simulink model "superProgramParameterObserving"  (R2014b)
settings: Solver=FixedStepDiscrete  StartTime=0.0  StopTime=10.0  RelTol=1e-3
libraries: c2833xlib x19, c280xlib x7, simulink x1
(part 2 of 2)

== stateflow chart superProgramParameterObserving/stackerController ==
  state stateOne [parallel]
    settings: executionOrder=10
    state storeValue
      entry: lightBarrierTriggeredValue = lightBarrierCrossed;
      colorSensorTriggeredValue = colorSensor;
    state idle
    state start
      entry: lightBarrierTriggeredValue = false;
      colorSensorTriggeredValue = uint16(9999);
    state wait
    stateOne.idle -> storeValue : after(0.01,msec)
    (default) -> stateOne.start
    stateOne.start -> stateOne.idle
    wait -> stateOne.idle
    storeValue -> wait : after(0.01,msec)
  state startingSequence [parallel]
    settings: executionOrder=1
    state prepareStacker
      entry:
      stackerMode = int16(0);
      speedCenterPivotTable = uint16(0);
      directionCenterPivotTable = true;
      speedTowerShifter = uint16(0);
      directionTowerShifter = true;
      speedDoorOpener = uint16(75);
      directionDoorOpener = false;
      paternosterSpeed_controller.setPaternosterSpeed(uint16(0));
      directionPaternoster = true;
      speedKicker = uint16(0);
      directionKicker = true;
      speedTipper = uint16(0);
      directionTipper = true;
      enableCounter;
      state prepareTipper [parallel]
        settings: executionOrder=1
        state tipperPreparation
          entry: directionTipper = true;
          speedTipper = tipperSpeed;
        state stopKickerInStartingPosition
          entry: speedTipper = uint16(0);
        (default) -> startingSequence.prepareStacker.prepareTipper.tipperPreparation
        startingSequence.prepareStacker.prepareTipper.tipperPreparation -> stopKickerInStartingPosition : [innerTipperButton == true]
      state prepareKicker [parallel]
        settings: executionOrder=2
        state startKickerMovement
          entry: speedKicker = uint16(100);
          directionKicker = true;
        state stopKickerMovement
          entry: speedKicker = uint16(0);
        startingSequence.prepareStacker.prepareKicker.startKickerMovement -> startingSequence.prepareStacker.prepareKicker.stopKickerMovement : [innerKickerButton == true]
        (default) -> startingSequence.prepareStacker.prepareKicker.startKickerMovement
      state shiftStackerAndOpenDoor [parallel]
        settings: executionOrder=3
        state blockTowerIdle
        state shiftTowerForwards
          entry: speedDoorOpener = uint16(0);
          directionTowerShifter = false;
          speedTowerShifter = towerShifterSpeed;
        state stopOpeningDoor
          entry: speedDoorOpener = uint16(0);
        state stopTowerShifting
          entry: speedTowerShifter = uint16(0);
          directionTowerShifter = true;
        state openDoor
          entry: directionDoorOpener = true;
          speedDoorOpener = uint16(70);
        blockTowerIdle -> shiftTowerForwards : [towerShifterButton == true]
        (default) -> blockTowerIdle
        shiftTowerForwards -> startingSequence.prepareStacker.shiftStackerAndOpenDoor.stopTowerShifting : [towerShifterButton == false]
        openDoor -> startingSequence.prepareStacker.shiftStackerAndOpenDoor.stopOpeningDoor : [towerShifterButton == false]
        startingSequence.prepareStacker.shiftStackerAndOpenDoor.stopTowerShifting -> openDoor : [towerShifterButton == true]
        startingSequence.prepareStacker.shiftStackerAndOpenDoor.stopOpeningDoor -> openDoor : [towerShifterButton == true]
      state emptyTipper [parallel]
        settings: executionOrder=4
        state wait_1
        state moveTipperIn
          entry: directionTipper = true;
        state tipperIdle
        state moveTipperOut
          entry: directionTipper = false;
          speedTipper = tipperSpeed;
        state wait_2
        (default) -> startingSequence.prepareStacker.emptyTipper.tipperIdle
        startingSequence.prepareStacker.emptyTipper.tipperIdle -> wait_1 : [[outerTipperButton == true] && [innerTipperButton == true]]
        wait_1 -> moveTipperOut : after(1300,msec)
        moveTipperOut -> moveTipperIn : [outerTipperButton == true]
        wait_2 -> startingSequence.prepareStacker.emptyTipper.tipperIdle : after(1300,msec)
        moveTipperIn -> moveTipperOut [order 2] : [innerTipperButton == true]
        moveTipperIn -> wait_2 [order 1] : [[outerTipperButton == true] && [innerTipperButton == true]]
    state operationMode
    state waitingForButtonRelaseToStartSuperProgram
    (default) -> prepareStacker
    prepareStacker -> waitingForButtonRelaseToStartSuperProgram : [powerButton == true]
    waitingForButtonRelaseToStartSuperProgram -> operationMode : [powerButton == false] {send(sorting.START); send(timer.START);}
  state timer [parallel]
    settings: executionOrder=2
    state startReturningBlocksFromRecervoir
      entry: send(sorting.STARTRESORTING);
    state start
    state inactive
    inactive -> startReturningBlocksFromRecervoir : after(latestPointInTimeToAcceptBlockDelivery,sec)
    (default) -> timer.start
    timer.start -> inactive : START
  state statusLED [parallel]
    settings: executionOrder=7
    state LED_1 [parallel]
      settings: executionOrder=1
      state off
        entry: statusLED_1 = false;
      state flash
        entry: statusLED_1 = true;
      state on
        entry: statusLED_1 = true;
      (default) -> statusLED.LED_1.off
      statusLED.LED_1.off -> statusLED.LED_1.on [order 1] : ON
      statusLED.LED_1.on -> statusLED.LED_1.off : OFF
      statusLED.LED_1.flash -> statusLED.LED_1.off : after(300,msec)
      statusLED.LED_1.off -> statusLED.LED_1.flash [order 2] : FLASH
    state LED_2 [parallel]
      settings: executionOrder=2
      state off
        entry: statusLED_2 = false;
      state flash
        entry: statusLED_2 = true;
      state on
        entry: statusLED_2 = true;
      (default) -> statusLED.LED_2.off
      statusLED.LED_2.off -> statusLED.LED_2.on [order 1] : ON
      statusLED.LED_2.on -> statusLED.LED_2.off : OFF
      statusLED.LED_2.flash -> statusLED.LED_2.off : after(300,msec)
      statusLED.LED_2.off -> statusLED.LED_2.flash [order 2] : FLASH
    state LED_3 [parallel]
      settings: executionOrder=3
      state off
        entry: statusLED_3 = false;
      state flash
        entry: statusLED_3 = true;
      state on
        entry: statusLED_3 = true;
      (default) -> statusLED.LED_3.off
      statusLED.LED_3.off -> statusLED.LED_3.on [order 1] : ON
      statusLED.LED_3.on -> statusLED.LED_3.off : OFF
      statusLED.LED_3.flash -> statusLED.LED_3.off : after(300,msec)
      statusLED.LED_3.off -> statusLED.LED_3.flash [order 2] : FLASH
    state LED_4 [parallel]
      settings: executionOrder=4
      state off
        entry: statusLED_4 = false;
      state flash
        entry: statusLED_4 = true;
      state on
        entry: statusLED_4 = true;
      (default) -> statusLED.LED_4.off
      statusLED.LED_4.off -> statusLED.LED_4.on [order 1] : ON
      statusLED.LED_4.on -> statusLED.LED_4.off : OFF
      statusLED.LED_4.flash -> statusLED.LED_4.off : after(300,msec)
      statusLED.LED_4.off -> statusLED.LED_4.flash [order 2] : FLASH
    state LED_finish [parallel]
      settings: executionOrder=5
      state off
        entry: LED_finish = false;
      state flash
        entry: LED_finish = true;
      state on
        entry: LED_finish = true;
      (default) -> statusLED.LED_finish.off
      statusLED.LED_finish.off -> statusLED.LED_finish.on [order 1] : ON
      statusLED.LED_finish.on -> statusLED.LED_finish.off : OFF
      statusLED.LED_finish.flash -> statusLED.LED_finish.off : after(300,msec)
      statusLED.LED_finish.off -> statusLED.LED_finish.flash [order 2] : FLASH
  state counterFromLightBarrierCrossed [parallel]
    settings: executionOrder=3
    state counter
      (history)
      state start
        entry: count = uint32(0);
      state highLevel
      state lowLevel
        entry: count = count + 1;
      counterFromLightBarrierCrossed.counter.lowLevel -> counterFromLightBarrierCrossed.counter.highLevel : [encoderPaternoster == true]
      (default) -> counterFromLightBarrierCrossed.counter.start
      counterFromLightBarrierCrossed.counter.start -> counterFromLightBarrierCrossed.counter.lowLevel : [encoderPaternoster == true]
      counterFromLightBarrierCrossed.counter.highLevel -> counterFromLightBarrierCrossed.counter.lowLevel : [encoderPaternoster == false]
      counterFromLightBarrierCrossed.counter -> counterFromLightBarrierCrossed.counter.start [order 1] : RESET
    state counting_off
    (default) -> counterFromLightBarrierCrossed.counter
    counterFromLightBarrierCrossed.counting_off -> counterFromLightBarrierCrossed.counter : [counterIsEnabled]
    counterFromLightBarrierCrossed.counter -> counterFromLightBarrierCrossed.counting_off [order 1] : [counterIsDisabled]
  state paternosterSpeed_controller [parallel]
    settings: executionOrder=4
    state moveToLastUnblockedPosition
      entry: directionPaternoster = true;
    state paternosterBlocked_errorRoutine
      entry: disableCounter;
      directionPaternoster = false;
      speedPaternoster = uint16(75);
    state restoreNormalPaternosterMode
    state counter
      entry: speedPaternoster = paternosterSpeed_controller.internalPaternosterSpeed;
      (history)
      state highLevel
      state lowLevel
      paternosterSpeed_controller.counter.lowLevel -> paternosterSpeed_controller.counter.highLevel [order 1] : [encoderPaternoster == true]
      (default) -> paternosterSpeed_controller.counter.lowLevel
      paternosterSpeed_controller.counter.highLevel -> paternosterSpeed_controller.counter.lowLevel [order 1] : [encoderPaternoster == false]
    paternosterSpeed_controller.counter.highLevel -> paternosterBlocked_errorRoutine [order 2] : [after(900,msec) && [paternosterSpeed_controller.internalPaternosterSpeed ~= 0]]
    paternosterBlocked_errorRoutine -> moveToLastUnblockedPosition : after(400,msec)
    moveToLastUnblockedPosition -> restoreNormalPaternosterMode : after(400,msec)
    paternosterSpeed_controller.counter.lowLevel -> paternosterBlocked_errorRoutine [order 2] : [after(900,msec) && [paternosterSpeed_controller.internalPaternosterSpeed ~= 0]]
    restoreNormalPaternosterMode -> paternosterSpeed_controller.counter : /{enableCounter;}
    (default) -> paternosterSpeed_controller.counter
    paternosterSpeed_controller.counter -> paternosterSpeed_controller.counter : UPDATEPATERNOSTERSPEED
  state stackerModeStatusLED_controller [parallel]
    settings: executionOrder=8
    state stackerPreparation
      entry: statusLED.LED_1.FLASH;
      statusLED.LED_2.FLASH;
      statusLED.LED_3.FLASH;
      statusLED.LED_4.FLASH;
    state waitingForFirstDelivery
      entry: statusLED.LED_1.ON;
      statusLED.LED_2.ON;
      statusLED.LED_3.ON;
      statusLED.LED_4.ON;
    state colorSortingFirstDelivery
      entry: statusLED.LED_1.ON;
    state waitingForSecondDelivery
      entry: statusLED.LED_2.ON;
    state changeMode
      entry: statusLED.LED_1.OFF;
      statusLED.LED_2.OFF;
      statusLED.LED_3.OFF;
      statusLED.LED_4.OFF;
    state colorSortingSecondDelivery
      entry: statusLED.LED_3.ON;
    state resorting
      entry: statusLED.LED_4.ON;
    state demolding
      entry: statusLED.LED_1.ON;
      statusLED.LED_2.ON;
      statusLED.LED_3.ON;
      statusLED.LED_4.ON;
    state finish
      entry: statusLED.LED_1.FLASH;
      statusLED.LED_2.FLASH;
      statusLED.LED_3.FLASH;
      statusLED.LED_4.FLASH;
    changeMode -> stackerPreparation [order 1] : [stackerMode == 0]
    stackerPreparation -> changeMode : after(1200,msec)
    changeMode -> stackerModeStatusLED_controller.waitingForFirstDelivery [order 2] : [stackerMode == 1]
    stackerModeStatusLED_controller.waitingForFirstDelivery -> changeMode : [stackerMode ~= 1]
    changeMode -> colorSortingFirstDelivery [order 3] : [stackerMode == 2]
    colorSortingFirstDelivery -> changeMode : [stackerMode ~= 2]
    changeMode -> stackerModeStatusLED_controller.waitingForSecondDelivery [order 6] : [stackerMode ==3]
    stackerModeStatusLED_controller.waitingForSecondDelivery -> changeMode : [stackerMode ~= 3]
    changeMode -> colorSortingSecondDelivery [order 4] : [stackerMode == 4]
    colorSortingSecondDelivery -> changeMode : [stackerMode ~= 4]
    (default) -> changeMode
    stackerModeStatusLED_controller.finish -> changeMode : after(600,msec)
    changeMode -> stackerModeStatusLED_controller.finish [order 8] : [stackerMode == 7]
    stackerModeStatusLED_controller.demolding -> changeMode : [stackerMode ~= 6]
    changeMode -> stackerModeStatusLED_controller.demolding [order 7] : [stackerMode == 6]
    resorting -> changeMode : [stackerMode ~= 5]
    changeMode -> resorting [order 5] : [stackerMode == 5]
  note: stackerModes:
      | 0: stackerPreparation
      | 1: waitingForFirstDelivery
      | 2: colorSortingFirstDelivery
      | 3: waitingForSecondDelivery
      | 4: colorSortingSecondDelivery
      | 5: resorting
      | 6: demolding
      | 7: finish
  state blockCounter [parallel]
    settings: executionOrder=9
    state start
      entry: blueBlocksPassed = uint16(0);
      redBlocksPassed = uint16(0);
    state idle
      entry: totalBlocksPassed = blueBlocksPassed + redBlocksPassed;
    blockCounter.idle -> blockCounter.idle [order 2] : ADDBLUEBLOCK
        | /{blueBlocksPassed = blueBlocksPassed + 1;
        | blueBlocksInRecervoir = blueBlocksInRecervoir + 1;}
    blockCounter.start -> blockCounter.idle
    (default) -> blockCounter.start : {blueBlocksInRecervoir = uint16(0);}
    blockCounter.idle -> blockCounter.idle [order 1] : ADDREDBLOCK
        | /{redBlocksPassed = redBlocksPassed + 1;}
    blockCounter -> blockCounter.start : RESET
  state stateTwo [parallel]
    settings: executionOrder=11
    state start
      entry: stateOne.lightBarrierTriggeredValue = stateOne.lightBarrierTriggeredValue;
      stateOne.colorSensorTriggeredValue = stateOne.colorSensorTriggeredValue;
    state end
      entry: stateOne.lightBarrierTriggeredValue = stateOne.lightBarrierTriggeredValue;
      stateOne.colorSensorTriggeredValue = stateOne.colorSensorTriggeredValue;
    (default) -> stateTwo.start
    stateTwo.start -> end
    end -> stateTwo.start : after(0.01,msec)
  state sorting [parallel]
    settings: executionOrder=6
    state resorting_controller
      entry: counterFromLightBarrierCrossed.counter.RESET;
      stackerMode = int16(5);
      blocksInChute = blocksInChute + abs(blocksInChute) * int16([blocksInChute < 0]);
      blocksToTip = int16(blockCapacityFromTipperToPaternosterIntake) - blocksInChute;
      paternosterSpeed_controller.setPaternosterSpeed(paternosterMaximumSpeed);
      state chuteEnquing_controller [parallel]
        settings: executionOrder=1
        state counterDisabled
        state chuteEnqueuing_controller
          (history)
          state idle
          state signalizeFreeSlotInChute
            exit: resorting_controller.blocksToTip = resorting_controller.blocksToTip + 1;
          sorting.resorting_controller.chuteEnquing_controller.chuteEnqueuing_controller.idle -> signalizeFreeSlotInChute : [lightBarrierCrossed == true]
              | {counterFromLightBarrierCrossed.counter.RESET;
              | send(blockCounter.ADDREDBLOCK);}
          (default) -> sorting.resorting_controller.chuteEnquing_controller.chuteEnqueuing_controller.idle
          signalizeFreeSlotInChute -> sorting.resorting_controller.chuteEnquing_controller.chuteEnqueuing_controller.idle : [lightBarrierCrossed == false]
        (default) -> counterDisabled
        chuteEnqueuing_controller -> counterDisabled : [counterIsDisabled]
        counterDisabled -> chuteEnqueuing_controller : [counterIsEnabled]
      state tipper_controller [parallel]
        settings: executionOrder=2
        state tip
          exit: resorting_controller.blocksToTip = resorting_controller. blocksToTip - 1;
          blockCounter.blueBlocksInRecervoir = blockCounter.blueBlocksInRecervoir - 1;
          state tipperMovement
            state tipperPreparation
              entry: directionTipper = false;
              speedTipper = tipperSpeed;
            state tipperBlocked_errorRoutine
              state waitForResolvingOfBlockage
                entry: speedTipper = uint16(0);
              state removeTipperFromBlockage
                entry: directionTipper = false;
                speedTipper = tipperSpeed;
              removeTipperFromBlockage -> waitForResolvingOfBlockage : [outerTipperButton == true]
              (default) -> removeTipperFromBlockage
            state tipperPush
              entry: directionTipper = true;
            state tipperRemove
              entry: directionTipper = false;
            state tipperIdle
              entry: speedTipper = uint16(0);
            (default) -> sorting.resorting_controller.tipper_controller.tip.tipperMovement.tipperPreparation
            waitForResolvingOfBlockage -> sorting.resorting_controller.tipper_controller.tip.tipperMovement.tipperPreparation : after(300,msec)
            sorting.resorting_controller.tipper_controller.tip.tipperMovement.tipperPreparation -> tipperPush : [outerTipperButton == true]
            tipperPush -> tipperBlocked_errorRoutine [order 2] : after(500,msec)
            tipperPush -> tipperRemove [order 1] : [innerTipperButton == true]
            tipperRemove -> sorting.resorting_controller.tipper_controller.tip.tipperMovement.tipperIdle : [outerTipperButton == true]
          (default) -> tipperMovement
        state tipperIdle
        sorting.resorting_controller.tipper_controller.tipperIdle -> tip : [resorting_controller.blocksToTip > 0]
        (default) -> sorting.resorting_controller.tipper_controller.tipperIdle
        sorting.resorting_controller.tipper_controller.tip.tipperMovement.tipperIdle -> sorting.resorting_controller.tipper_controller.tipperIdle : after(250,msec)
    state colorSorter
      entry: paternosterSpeed_controller.setPaternosterSpeed(paternosterSpeed);
      state counterFromKick [parallel]
        settings: executionOrder=2
        state counter
          (history)
          state start
            entry: count = uint32(0);
          state highLevel
          state lowLevel
            entry: count = count + 1;
          sorting.colorSorter.counterFromKick.counter.lowLevel -> sorting.colorSorter.counterFromKick.counter.highLevel : [encoderPaternoster == true]
          (default) -> sorting.colorSorter.counterFromKick.counter.start
          sorting.colorSorter.counterFromKick.counter.start -> sorting.colorSorter.counterFromKick.counter.lowLevel : [encoderPaternoster == true]
          sorting.colorSorter.counterFromKick.counter.highLevel -> sorting.colorSorter.counterFromKick.counter.lowLevel : [encoderPaternoster == false]
          sorting.colorSorter.counterFromKick.counter -> sorting.colorSorter.counterFromKick.counter.start [order 1] : RESET
        state counting_off
        sorting.colorSorter.counterFromKick.counting_off -> sorting.colorSorter.counterFromKick.counter : [counterIsEnabled]
        (default) -> sorting.colorSorter.counterFromKick.counting_off
        sorting.colorSorter.counterFromKick.counter -> sorting.colorSorter.counterFromKick.counting_off [order 1] : [counterIsDisabled]
      state kicker [parallel]
        settings: executionOrder=1
        state kicker_controller [parallel]
          settings: executionOrder=1
          state kick
            entry: send(colorSorter.counterFromKick.counter.RESET);
            enqueuedBlocksToKick = enqueuedBlocksToKick -1;
            state startKickerMovement
              entry: directionKicker = false;
              speedKicker = uint16(100);
            state stopKickerMovement
              entry: speedKicker = uint16(0);
            state kickerBlocked_errorRoutine
              state dissolveBlockage
                entry: disableCounter;
                paternosterSpeed_controller.setPaternosterSpeed(uint16(70));
                directionPaternoster = false;
              state resumeNormalPaternosterOperatingMode
                exit: enableCounter;
                directionPaternoster = true;
                speedPaternoster = uint16(paternosterSpeed);
              (default) -> sorting.colorSorter.kicker.kicker_controller.kick.kickerBlocked_errorRoutine.dissolveBlockage
              sorting.colorSorter.kicker.kicker_controller.kick.kickerBlocked_errorRoutine.dissolveBlockage -> sorting.colorSorter.kicker.kicker_controller.kick.kickerBlocked_errorRoutine.resumeNormalPaternosterOperatingMode : [outerKickerButton == true]
            sorting.colorSorter.kicker.kicker_controller.kick.startKickerMovement -> sorting.colorSorter.kicker.kicker_controller.kick.stopKickerMovement [order 1] : [outerKickerButton == true]
            (default) -> sorting.colorSorter.kicker.kicker_controller.kick.startKickerMovement
            sorting.colorSorter.kicker.kicker_controller.kick.kickerBlocked_errorRoutine.resumeNormalPaternosterOperatingMode -> sorting.colorSorter.kicker.kicker_controller.kick.stopKickerMovement
            sorting.colorSorter.kicker.kicker_controller.kick.startKickerMovement -> sorting.colorSorter.kicker.kicker_controller.kick.kickerBlocked_errorRoutine [order 2] : after(kickerBlockedTimeout,msec)
          state idle
            entry: speedKicker = uint16(0);
          state reprepareKicker
            state kickerBlocked_errorRoutine
              state dissolveBlockage
                entry: speedKicker = uint16(100);
                directionKicker = false;
              (default) -> sorting.colorSorter.kicker.kicker_controller.reprepareKicker.kickerBlocked_errorRoutine.dissolveBlockage
            state startKickerMovement
              entry: speedKicker = uint16(100);
              directionKicker = true;
            state stopKickerMovement
              entry: speedKicker = uint16(0);
            sorting.colorSorter.kicker.kicker_controller.reprepareKicker.startKickerMovement -> sorting.colorSorter.kicker.kicker_controller.reprepareKicker.kickerBlocked_errorRoutine [order 2] : after(kickerBlockedTimeout,msec)
            sorting.colorSorter.kicker.kicker_controller.reprepareKicker.kickerBlocked_errorRoutine.dissolveBlockage -> sorting.colorSorter.kicker.kicker_controller.reprepareKicker.startKickerMovement : [outerKickerButton == true]
            sorting.colorSorter.kicker.kicker_controller.reprepareKicker.startKickerMovement -> sorting.colorSorter.kicker.kicker_controller.reprepareKicker.stopKickerMovement [order 1] : [innerKickerButton == true]
            (default) -> sorting.colorSorter.kicker.kicker_controller.reprepareKicker.startKickerMovement
          (default) -> sorting.colorSorter.kicker.kicker_controller.idle
          sorting.colorSorter.kicker.kicker_controller.idle -> kick : [[counterFromLightBarrierCrossed.counter.count >= positionOfStartingKickOut] && [enqueuedBlocksToKick > 0]]
          kick -> reprepareKicker : [colorSorter.counterFromKick.counter.count >= freeSpaceTillReprepareKickerAfterKickOut]
          sorting.colorSorter.kicker.kicker_controller.reprepareKicker.stopKickerMovement -> sorting.colorSorter.kicker.kicker_controller.idle
      state lightBarrier_controller [parallel]
        settings: executionOrder=3
        state controller
          (history)
          state lightBarrierCrossed
            entry:
            send(colorSorter.color_controller.controller.NEXTBLOCK);
          state idle
          state waitngForSecondMeasuring
            entry: send(counterFromLightBarrierCrossed.counter.RESET);
          state secondMeasuring
          (default) -> sorting.colorSorter.lightBarrier_controller.controller.idle : /{colorSorter.kicker.kicker_controller.enqueuedBlocksToKick =uint16( 0)}
          sorting.colorSorter.lightBarrier_controller.controller.idle -> waitngForSecondMeasuring : [lightBarrierCrossed  == true]
          waitngForSecondMeasuring -> secondMeasuring : [counterFromLightBarrierCrossed.counter.count >= 11]
          secondMeasuring -> lightBarrierCrossed [order 1] : [lightBarrierCrossed == true]
          secondMeasuring -> (junction 743) [order 2] : [lightBarrierCrossed == false]
          lightBarrierCrossed -> (junction 743) : [lightBarrierCrossed == false]
          (junction 743) -> sorting.colorSorter.lightBarrier_controller.controller.idle
        state controller_off
        sorting.colorSorter.lightBarrier_controller.controller_off -> sorting.colorSorter.lightBarrier_controller.controller : [counterIsEnabled]
        (default) -> sorting.colorSorter.lightBarrier_controller.controller_off
        sorting.colorSorter.lightBarrier_controller.controller -> sorting.colorSorter.lightBarrier_controller.controller_off : [counterIsDisabled]
      state color_controller [parallel]
        settings: executionOrder=4
        state controller
          (history)
          note: blue block detected
          state blockToKick
            entry: colorSorter.kicker.kicker_controller.enqueuedBlocksToKick = colorSorter.kicker.kicker_controller.enqueuedBlocksToKick + 1;
          state blockNotToKick
          state waitingForBlockToPassColorSensor
          note: red block detected
          (default) -> blockNotToKick
          waitingForBlockToPassColorSensor -> (junction 782) [order 1] : [counterFromLightBarrierCrossed.counter.count >= lastPositionToDetectBlockColor]
          (junction 782) -> blockToKick [order 1] : [shouldBeKicked == true]
              | /{send(blockCounter.ADDBLUEBLOCK);}
          blockNotToKick -> waitingForBlockToPassColorSensor : NEXTBLOCK /{shouldBeKicked = true;}
          (junction 782) -> (junction 783) [order 2] : [shouldBeKicked == false]
              | /{send(blockCounter.ADDREDBLOCK);}
          waitingForBlockToPassColorSensor -> waitingForBlockToPassColorSensor [order 2] : [colorSensor <= colorSorterBlockColorLimit] {shouldBeKicked = false;}
          (junction 783) -> blockNotToKick
          blockToKick -> (junction 783)
        state controller_off
        sorting.colorSorter.color_controller.controller_off -> sorting.colorSorter.color_controller.controller : [counterIsEnabled]
        (default) -> sorting.colorSorter.color_controller.controller_off
        sorting.colorSorter.color_controller.controller -> sorting.colorSorter.color_controller.controller_off : [counterIsDisabled]
    state prepareKickerAsWall
      state startKickerMovement
        entry: directionKicker = false;
        speedKicker = uint16(100);
      state stopKickerMovement
        entry: speedKicker = uint16(0);
      state kickerBlocked_errorRoutine
        state dissolveBlockage
          entry: disableCounter;
          paternosterSpeed_controller.setPaternosterSpeed(uint16(70));
          directionPaternoster = false;
        state resumeNormalPaternosterOperatingMode
          exit: enableCounter;
          directionPaternoster = true;
          speedPaternoster = uint16(paternosterSpeed);
        (default) -> sorting.prepareKickerAsWall.kickerBlocked_errorRoutine.dissolveBlockage
        sorting.prepareKickerAsWall.kickerBlocked_errorRoutine.dissolveBlockage -> sorting.prepareKickerAsWall.kickerBlocked_errorRoutine.resumeNormalPaternosterOperatingMode : [outerKickerButton == true]
      sorting.prepareKickerAsWall.startKickerMovement -> sorting.prepareKickerAsWall.stopKickerMovement [order 1] : [outerKickerButton == true]
      (default) -> sorting.prepareKickerAsWall.startKickerMovement
      sorting.prepareKickerAsWall.kickerBlocked_errorRoutine.resumeNormalPaternosterOperatingMode -> sorting.prepareKickerAsWall.stopKickerMovement
      sorting.prepareKickerAsWall.startKickerMovement -> sorting.prepareKickerAsWall.kickerBlocked_errorRoutine [order 2] : after(kickerBlockedTimeout,msec)
    state waitingForBlocksToReachTower
      state blockReachedTopOfPaternoster
        entry: paternosterSpeed_controller.setPaternosterSpeed(uint16(0));
      state allBlocksFallenIntoTower
      state start
      (default) -> sorting.waitingForBlocksToReachTower.start
      blockReachedTopOfPaternoster -> allBlocksFallenIntoTower : after(timeBlockNeedsToFallIntoTowerFromTopOfPaternoster,msec)
      sorting.waitingForBlocksToReachTower.start -> blockReachedTopOfPaternoster
    state waitingForBlocksToReachTDCOfPaternoster_1
    state finish
      entry: stackerMode = int16(7);
      statusLED.LED_finish.ON;
    state demolding
      entry: stackerMode = int16(6);
      state doorOpening
        state stopOpeningDoor
          entry: speedDoorOpener = uint16(0);
        state startOpeningDoor
          entry: directionDoorOpener = true;
          speedDoorOpener = uint16(90);
        (default) -> startOpeningDoor
        startOpeningDoor -> sorting.demolding.doorOpening.stopOpeningDoor : after(850,msec)
      state towerShifting
        state stopTowerShifting
          entry: speedTowerShifter = uint16(0);
        state startTowerShifting
          entry: speedTowerShifter = towerShifterSpeed;
        startTowerShifting -> sorting.demolding.towerShifting.stopTowerShifting : [towerShifterButton == true]
        (default) -> startTowerShifting
      sorting.demolding.doorOpening.stopOpeningDoor -> towerShifting : after(400,msec)
      (default) -> doorOpening
    state stackerPositioning
      state stackerRotationMovement [parallel]
        settings: executionOrder=1
        state targetAngleReached
          entry: speedCenterPivotTable = uint16(0);
        state rotationMovement
          entry: send(sorting.stackerPositioning.counterCenterPivotTable.RESET);
          directionCenterPivotTable = false;
          speedCenterPivotTable =centerPivotTableSpeed;
          targetTics = centerPivotTableRotationTargetAngle / 360 * 75 * centerPivotTableTransitionRatio;
        sorting.stackerPositioning.stackerRotationMovement.rotationMovement -> sorting.stackerPositioning.stackerRotationMovement.targetAngleReached : [sorting.stackerPositioning.counterCenterPivotTable.count >= targetTics]
        (default) -> sorting.stackerPositioning.stackerRotationMovement.rotationMovement
      state counterCenterPivotTable [parallel]
        settings: executionOrder=2
        state start
          entry: count = uint32(0);
        state highLevel
          entry: count = count + 1;
        state lowLevel
        sorting.stackerPositioning.counterCenterPivotTable.highLevel -> sorting.stackerPositioning.counterCenterPivotTable.lowLevel : [encoderCenterPivotTable == true]
        (default) -> sorting.stackerPositioning.counterCenterPivotTable.start
        sorting.stackerPositioning.counterCenterPivotTable.start -> sorting.stackerPositioning.counterCenterPivotTable.highLevel : [encoderCenterPivotTable == true]
        sorting.stackerPositioning.counterCenterPivotTable.lowLevel -> sorting.stackerPositioning.counterCenterPivotTable.highLevel : [encoderCenterPivotTable == false]
        sorting.stackerPositioning.counterCenterPivotTable -> sorting.stackerPositioning.counterCenterPivotTable.start : RESET
    state stackerRotation
      state stackerRotationMovement [parallel]
        settings: executionOrder=1
        state targetAngleReached
          entry: speedCenterPivotTable = uint16(0);
        state rotationMovement
          entry: send(sorting.stackerRotation.counterCenterPivotTable.RESET);
          directionCenterPivotTable = true;
          speedCenterPivotTable =centerPivotTableSpeed;
          targetTics = centerPivotTableRotationTargetAngle / 360 * 75 * centerPivotTableTransitionRatio;
        sorting.stackerRotation.stackerRotationMovement.rotationMovement -> sorting.stackerRotation.stackerRotationMovement.targetAngleReached : [sorting.stackerRotation.counterCenterPivotTable.count >= targetTics]
        (default) -> sorting.stackerRotation.stackerRotationMovement.rotationMovement
      state counterCenterPivotTable [parallel]
        settings: executionOrder=2
        state start
          entry: count = uint32(0);
        state highLevel
          entry: count = count + 1;
        state lowLevel
        sorting.stackerRotation.counterCenterPivotTable.highLevel -> sorting.stackerRotation.counterCenterPivotTable.lowLevel : [encoderCenterPivotTable == true]
        (default) -> sorting.stackerRotation.counterCenterPivotTable.start
        sorting.stackerRotation.counterCenterPivotTable.start -> sorting.stackerRotation.counterCenterPivotTable.highLevel : [encoderCenterPivotTable == true]
        sorting.stackerRotation.counterCenterPivotTable.lowLevel -> sorting.stackerRotation.counterCenterPivotTable.highLevel : [encoderCenterPivotTable == false]
        sorting.stackerRotation.counterCenterPivotTable -> sorting.stackerRotation.counterCenterPivotTable.start : RESET
    state waitingForFirstDelivery
    state start
    state waitingForBlocksToReachTDCOfPaternoster_2
    colorSorter -> prepareKickerAsWall [order 2] : [[stackerMode == 4] && [blockCounter.redBlocksPassed == 1]]
        | {resorting_controller.blocksInChute =  int16(6  - blockCounter.totalBlocksPassed);
        | blockCounter.maxBlueBlocksInRecervoir = blockCounter.blueBlocksInRecervoir;
        | blockCounter.maxBlocksLeftFromSecondDelivery =  uint16(6) - blockCounter.totalBlocksPassed;
        | send(blockCounter.RESET);}
    colorSorter -> prepareKickerAsWall [order 1] : [[stackerMode == 4] && [counterFromLightBarrierCrossed.counter.count >= ((toleratedBlocksForNotChangingStackerMode * distanceBetweenBlockHooks) + 14 * 3.75)]]
        | {resorting_controller.blocksInChute = int16(0);
        | blockCounter.maxBlueBlocksInRecervoir = blockCounter.blueBlocksInRecervoir;
        | blockCounter.maxBlocksLeftFromSecondDelivery = uint16(0);
        | send(blockCounter.RESET);}
    waitingForBlocksToReachTDCOfPaternoster_1 -> waitingForBlocksToReachTower : [counterFromLightBarrierCrossed.counter.count >= distanceFromLightBarrierToTDCOfPaternoster]
    resorting_controller -> waitingForBlocksToReachTDCOfPaternoster_1 [order 1] : [blockCounter.totalBlocksPassed >= (blockCounter.maxBlueBlocksInRecervoir + blockCounter.maxBlocksLeftFromSecondDelivery)]
    colorSorter -> prepareKickerAsWall [order 3] : STARTRESORTING {resorting_controller.blocksInChute = int16(0);}
    sorting.waitingForFirstDelivery -> colorSorter
    sorting.start -> stackerPositioning : START
    (default) -> sorting.start
    resorting_controller -> waitingForBlocksToReachTDCOfPaternoster_2 [order 2] : [counterFromLightBarrierCrossed.counter.count >= ( toleratedBlocksForNotChangingStackerMode * distanceBetweenBlockHooks)]
    waitingForBlocksToReachTDCOfPaternoster_2 -> waitingForBlocksToReachTower : [counterFromLightBarrierCrossed.counter.count >= max(distanceFromLightBarrierToTDCOfPaternoster, (toleratedBlocksForNotChangingStackerMode * distanceBetweenBlockHooks))]
    sorting.prepareKickerAsWall.stopKickerMovement -> resorting_controller
    sorting.demolding.towerShifting.stopTowerShifting -> stackerRotation
    sorting.stackerRotation.stackerRotationMovement.targetAngleReached -> sorting.finish
    sorting.stackerPositioning.stackerRotationMovement.targetAngleReached -> sorting.waitingForFirstDelivery
    allBlocksFallenIntoTower -> sorting.demolding
  state mode_controller [parallel]
    settings: executionOrder=5
    state waitingForSecondDelivery
      entry: stackerMode = int16(3);
      send(blockCounter.RESET);
    state firstDelivery
      entry: stackerMode = int16(2);
    state start
    state secondDelivery
      entry: stackerMode = int16(4);
    firstDelivery -> mode_controller.waitingForSecondDelivery : [counterFromLightBarrierCrossed.counter.count >= (minFreeHooksToChangeModeToWaitingForSecondDelivery * distanceBetweenBlockHooks)]
    mode_controller.waitingForSecondDelivery -> secondDelivery : [blockCounter.totalBlocksPassed >= 1]
    mode_controller.start -> firstDelivery : [blockCounter.totalBlocksPassed >= 1]
    (default) -> mode_controller.start
  data: lightBarrierTriggeredValue local boolean; colorSensorTriggeredValue local uint16 [0..]; count local uint32; speedToSet function_input; internalPaternosterSpeed local uint16 [0..100]; blueBlocksPassed local uint16 [0..]; redBlocksPassed local uint16 [0..]; blueBlocksInRecervoir local uint16 [0..]; totalBlocksPassed local uint16 [0..]; maxBlueBlocksInRecervoir local uint16 [0..]; maxBlocksLeftFromSecondDelivery local uint16 [0..]; counterStatus function_output; counterStatus function_output; blocksInChute local int16; blocksToTip local int16 [-6..15]; count local uint32; enqueuedBlocksToKick local uint16 [0..2]; shouldBeKicked local boolean; targetTics local single [0..]; count local uint32 [0..]; targetTics local single [0..]; count local uint32 [0..]; powerButton input boolean; paternosterSpeed input uint16 [0..100]; paternosterMaximumSpeed input uint16 [0..100]; centerPivotTableTransitionRatio input single [0..]; centerPivotTableSpeed input uint16 [0..100]; centerPivotTableRotationTargetAngle input single [-360..360]; encoderCenterPivotTable input boolean; latestPointInTimeToAcceptBlockDelivery input uint16 [0..]; speedDoorOpener output uint16 [0..100]; directionDoorOpener output boolean; speedTowerShifter output uint16 [0..100]; directionTowerShifter output boolean; speedCenterPivotTable output uint16 [0..100]; directionCenterPivotTable output boolean; speedPaternoster output uint16 [0..100]; directionPaternoster output boolean; speedKicker output uint16 [0..100]; directionKicker output boolean; speedTipper output uint16 [0..100]; directionTipper output boolean; encoderPaternoster input boolean; towerShifterButton input boolean; lightBarrierCrossed input boolean; colorSensor input uint16 [0..4095]; colorSorterBlockColorLimit input uint16 [0..4095]; lastPositionToDetectBlockColor input uint32; positionOfStartingKickOut input uint32; distanceBetweenBlockHooks input uint16 [0..]; towerShifterSpeed input uint16 [0..100]; distanceFromLightBarrierToTDCOfPaternoster input uint16 [0..]; freeSpaceTillReprepareKickerAfterKickOut input uint32; minFreeHooksToChangeModeToWaitingForSecondDelivery input uint16 [0..]; toleratedBlocksForNotChangingStackerMode input uint16 [0..]; kickerBlockedTimeout input uint16 [0..]; statusLED_1 output boolean; statusLED_2 output boolean; statusLED_3 output boolean; blockCapacityFromTipperToPaternosterIntake input uint16 [0..]; timeBlockNeedsToFallIntoTowerFromTopOfPaternoster input uint16 [0..]; outerTipperButton input boolean; innerTipperButton input boolean; tipperSpeed input uint16 [0..100]; stackerMode local int16; statusLED_4 output boolean; outerKickerButton input boolean; innerKickerButton input boolean; LED_finish output boolean; counterActivity local boolean
  data centerPivotTableTransitionRatio settings: description=transition ration of the stacker center pivot plate
  data centerPivotTableRotationTargetAngle settings: description=rotation target angle for the center pivot table of the stacker
  data encoderCenterPivotTable settings: description=encoder signal of the center pivot table motor
  data speedDoorOpener settings: description=speedCenterPivotTable of the center pivot table motor
  data directionDoorOpener settings: description=direciton of the center pivot table motor
  data speedTowerShifter settings: description=speedCenterPivotTable of the center pivot table motor
  data directionTowerShifter settings: description=direciton of the center pivot table motor
  data speedCenterPivotTable settings: description=speedCenterPivotTable of the center pivot table motor
  data directionCenterPivotTable settings: description=direciton of the center pivot table motor
  data directionPaternoster settings: description=direciton of the center pivot table motor
  data directionKicker settings: description=direciton of the center pivot table motor
  data directionTipper settings: description=direciton of the center pivot table motor
  data encoderPaternoster settings: description=encoder signal from the paternoster
  data towerShifterButton settings: description=encoder signal from the kicker
  data lightBarrierCrossed settings: description=bolean value if the light barrier is currently crossed
  data colorSensor settings: description=value from the ADC of the color sensor
  data colorSorterBlockColorLimit settings: description=color value limit between red and blue blocks which decides whether blocks should be kicked or not
  data lastPositionToDetectBlockColor settings: description=length from light barrier to last possible position for color detection of blocks in tics from encoder
  data positionOfStartingKickOut settings: description=length from light barrier to position where kicker starts off kicking out blocks in tics from encoder
  data freeSpaceTillReprepareKickerAfterKickOut settings: description=space to wait after the kick out of a block till kicker reprepares (crosses the drive lane again) in tics from encoder
  data kickerBlockedTimeout settings: description=distance to move kicker in / out
  data statusLED_1 settings: description=status LED to signalize when the light barrier is currently crossed
  events: START local FUNCTION_CALL_EVENT; FLASH local FUNCTION_CALL_EVENT; ON local FUNCTION_CALL_EVENT; OFF local FUNCTION_CALL_EVENT; FLASH local FUNCTION_CALL_EVENT; ON local FUNCTION_CALL_EVENT; OFF local FUNCTION_CALL_EVENT; FLASH local FUNCTION_CALL_EVENT; ON local FUNCTION_CALL_EVENT; OFF local FUNCTION_CALL_EVENT; FLASH local FUNCTION_CALL_EVENT; ON local FUNCTION_CALL_EVENT; OFF local FUNCTION_CALL_EVENT; FLASH local FUNCTION_CALL_EVENT; ON local FUNCTION_CALL_EVENT; OFF local FUNCTION_CALL_EVENT; RESET local FUNCTION_CALL_EVENT; UPDATEPATERNOSTERSPEED local FUNCTION_CALL_EVENT; RESET local FUNCTION_CALL_EVENT; ADDBLUEBLOCK local FUNCTION_CALL_EVENT; ADDREDBLOCK local FUNCTION_CALL_EVENT; RESET local FUNCTION_CALL_EVENT; NEXTBLOCK local FUNCTION_CALL_EVENT; RESET local FUNCTION_CALL_EVENT; RESET local FUNCTION_CALL_EVENT; STARTRESORTING local FUNCTION_CALL_EVENT; START local FUNCTION_CALL_EVENT
  function setPaternosterSpeed(speedToSet):
    | function setPaternosterSpeed(speedToSet)
    | %#codegen
    | internalPaternosterSpeed = speedToSet;
    | send(paternosterSpeed_controller.UPDATEPATERNOSTERSPEED);
  function disableCounter:
    | function disableCounter
    | %#codegen
    | counterActivity = false;
  function enableCounter:
    | function enableCounter
    | %#codegen
    | counterActivity =true;
  function counterStatus = counterIsEnabled:
    | function counterStatus = counterIsEnabled
    | %#codegen
    | if counterActivity == true
    |     counterStatus = true;
    | else
    |     counterStatus = false;
    | end
  function counterStatus = counterIsDisabled:
    | function counterStatus = counterIsDisabled
    | %#codegen
    | if counterActivity == false
    |     counterStatus = true;
    | else
    |     counterStatus = false;
    | end
